simulink model "Three_Level_Inverter"  (R2020b)
settings: Solver=VariableStepAuto  StartTime=0.0  StopTime=0.02  FixedStep=1e-9  RelTol=1e-3
values from neighbouring files (symbols this model uses):
  Tri_wave_dt = 25e-6    (= 2.5e-05)    [inv_sim.m]
  Ts = 2e-6    (= 2e-06)    [inv_sim.m]
libraries: ee_lib x55, fl_lib x36, nesl_utility x34, simulink x2
(part 1 of 2)
settings Model: Creator=ge62gas  LastModifiedBy=ge62gas

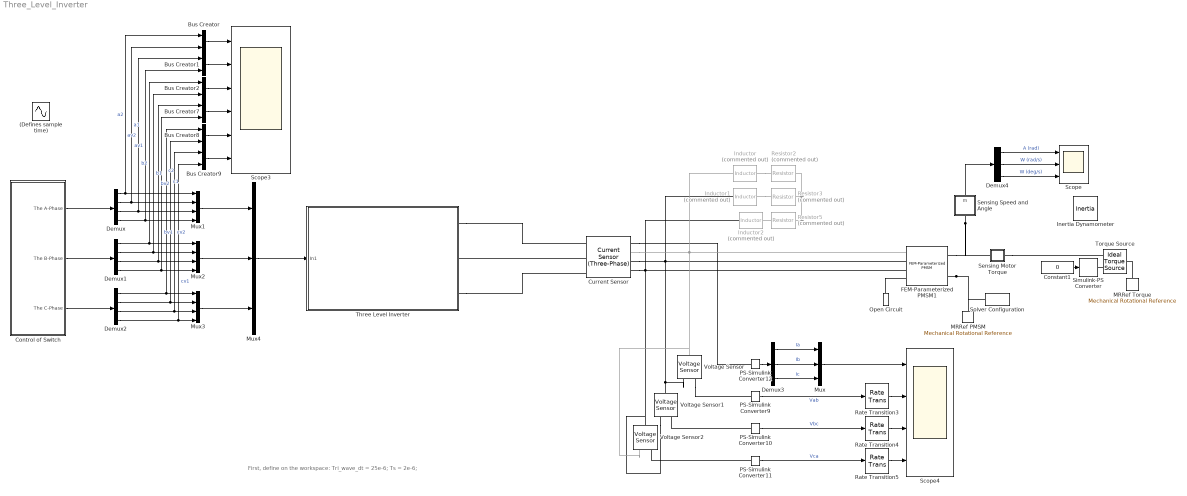
== system Three_Level_Inverter ==
  note: First, define on the workspace:
      |
      | Tri_wave_dt = 25e-6;
      | Ts = 2e-6;
  (Defines sample time) : Sin  SampleTime=Tri_wave_dt/10
  Bus Creator{,1..2,7..9} (6 alike) : BusCreator  Inputs=2
  Constant1 : Constant  Value=0
  Control of Switch : Subsystem
  Current Sensor : ee_lib/Sensors & Transducers/Current Sensor (Three-Phase)
      settings: SourceProductName=Electrical  InternalSimscapePortConfiguration="{\"Bottom\":[],\"Left\":[{\"id\":\"a1\",\"label\":\"a1\",\"type\":\"foundation.electrical.electrical\"},{\"id\":\"b1\",\"label\":\"b1\",\"type\":\"foundation.electrical.electrical\"},{\"id\":\"c1\",\"label\":\"c1\",\"type\":\"foundation.electrical.electrical\"}],\"Right\":[{\"id\":\"I_output\",\"label\":\"I\",\"type\":\"output\"},{\"id\":\"a2\",\"label\":\"a2\",\"type\":\"foundation.electrical.electrical\"},{\"id\":\"b2\",\"label\":\"b2\",\"type\":\"foundation.electrical.electrical\"},{\"id\":\"c2\",\"label\":\"c2\",\"type\":\"foundation.electrical.electrical\"}],\"Top\":[]}"
  Demux : Demux
  Demux1 : Demux
  Demux2 : Demux
  Demux3 : Demux  Outputs=3
  Demux4 : Demux  Outputs=3
  FEM-Parameterized PMSM1 : ee_lib/Electromechanical/Permanent Magnet/FEM-Parameterized PMSM  parameterization=1  winding_type=ee.enum.statorconnection.wye  iVec=[-2, 0, 2] A  xVec=xVec rad  dfluxdiMatrix=0.0002 * ones(3, 4) Wb/A  dfluxdxMatrix=[0, -.16, .16, 0; 0, -.16, .16, 0; 0, -.16, .16, 0] Wb/rad  calculate_torque_matrix=1  TorqueMatrix=zeros(3, 3, 3, 4) N*m  idVec1=[-200, 0, 200] A  iqVec1=[-200, 0, 200] A  LdMatrix=0.0002 * ones(3, 3) H  LqMatrix=0.0002 * ones(3, 3) H  PmMatrix=0.1 * ones(3, 3) Wb  N=6  interp_method=simscape.enum.interpolation.smooth  Rs=Rs Ohm  Ms=0.00002 H  L0=0.00016 H  losses_oc=[500 1500 0] W  losses_sc=[200 600 0] W  f_losses=140 Hz  Isc_losses=350 A  Inertia=0.01 kg*m^2  lam=0 N*m/(rad/s)  i_d_specify=on  i_d_priority=High  i_d=0 A  i_d_nominal_specify=off  i_d_nominal_unit=A  i_d_nominal_value=1  i_q_specify=on  i_q_priority=High  i_q=0 A  i_q_nominal_specify=off  i_q_nominal_unit=A  i_q_nominal_value=1  torque_specify=off  torque_priority=None  torque=0 N*m  torque_nominal_specify=off  torque_nominal_unit=N*m  torque_nominal_value=1  angular_velocity_specify=on  angular_velocity_priority=High  angular_velocity=3000 deg/s  angular_velocity_nominal_specify=off  angular_velocity_nominal_unit=rpm  angular_velocity_nominal_value=1  angular_position_specify=on  angular_position_priority=High  angular_position=11 deg  angular_position_nominal_specify=off  angular_position_nominal_unit=deg  angular_position_nominal_value=1  Tmeas=298.15 K  alpha=3.93e-3 1/K  alpha_flux=-0.001 1/K  stator_thermal_mass=100 J/K  stator_initial_temperatures=[298.15, 298.15, 298.15] K  rotor_thermal_mass=200 J/K  rotor_initial_temperature=298.15 K  Rm_percent_rotor=90  Rd_percent_rotor=30  idVec=idVec A  iqVec=iqVec A  dfluxAdiaMatrix3D=dfluxAdiaMatrix Wb/A  dfluxAdibMatrix3D=dfluxAdibMatrix Wb/A  dfluxAdicMatrix3D=dfluxAdicMatrix Wb/A  dfluxAdxMatrix3D=dfluxAdxMatrix Wb/rad  TorqueMatrix3D=TorqueMatrix N*m  iaVec=[-200, 0, 200] A  ibVec=[-200, 0, 200] A  icVec=[-200, 0, 200] A  dfluxAdiaMatrix=zeros(3, 3, 3, 4) Wb/A  dfluxAdibMatrix=zeros(3, 3, 3, 4) Wb/A  dfluxAdicMatrix=zeros(3, 3, 3, 4) Wb/A  dfluxAdxMatrix=zeros(3, 3, 3, 4) Wb/rad  param_dq0=1  winding_type_dq0=1  nPolePairs=4  parks_type=1  idVec2=[-200, 0, 200] A  iqVec2=[-200, 0, 200] A  magVec2=[0, 100, 200] A  betaVec2=[-180, -90, 0, 90, 180] deg  xVec2=[0, 5, 10, 15, 20, 25, 30] deg  fluxD_dq0=zeros(3, 3, 7) Wb  fluxQ_dq0=zeros(3, 3, 7) Wb  fluxA_dq0=zeros(3, 3, 7) Wb  Torque_dq0=zeros(3, 3, 7) N*m  fluxD_IBX=zeros(3, 5, 7) Wb  fluxQ_IBX=zeros(3, 5, 7) Wb  fluxA_IBX=zeros(3, 5, 7) Wb  Torque_IBX=zeros(3, 5, 7) N*m
      settings: SourceProductName=Electrical  LogSimulationData=on  InternalSimscapePortConfiguration="{\"Bottom\":[],\"Left\":[{\"id\":\"a\",\"label\":\"a\",\"type\":\"foundation.electrical.electrical\"},{\"id\":\"b\",\"label\":\"b\",\"type\":\"foundation.electrical.electrical\"},{\"id\":\"c\",\"label\":\"c\",\"type\":\"foundation.electrical.electrical\"},{\"id\":\"n\",\"label\":\"n\",\"type\":\"foundation.electrical.electrical\"}],\"Right\":[{\"id\":\"R\",\"label\":\"R\",\"type\":\"foundation.mechanical.rotational.rotational\"},{\"id\":\"C\",\"label\":\"C\",\"type\":\"foundation.mechanical.rotational.rotational\"}],\"Top\":[]}"
  Inductor : ee_lib/Passive/Inductor  Commented=on  l=1e-3 H  L_tol=20  enable_L_tol=0  tol_distribution=1  nSigma=4  r=0 Ohm  g=1e-9 1/Ohm  enable_operating_limits=0  operating_limit_action=2  max_working_current=1 A  power_rating=1 W  enable_faults=0  fault_action=1  lambdaPercent=50  k_faulted=0.9999  turnsShort=0  openCct=0  groundShort=0  groundShortG=0 1/Ohm  tau_fault=1e-3 s  enable_temporal_fault=0  t_fault=1 s  enable_behavioral_fault=0  max_permissible_voltage=100 V  n_fail_on_voltage=1  max_permissible_current=1 A  t_fail_on_current=1 s  i_L_specify=on  i_L_priority=High  i_L=-26 A  i_L_nominal_specify=off  i_L_nominal_unit=A  i_L_nominal_value=1
  Inductor1 : ee_lib/Passive/Inductor  Commented=on  l=1e-3 H  L_tol=20  enable_L_tol=0  tol_distribution=1  nSigma=4  r=0 Ohm  g=1e-9 1/Ohm  enable_operating_limits=0  operating_limit_action=2  max_working_current=1 A  power_rating=1 W  enable_faults=0  fault_action=1  lambdaPercent=50  k_faulted=0.9999  turnsShort=0  openCct=0  groundShort=0  groundShortG=0 1/Ohm  tau_fault=1e-3 s  enable_temporal_fault=0  t_fault=1 s  enable_behavioral_fault=0  max_permissible_voltage=100 V  n_fail_on_voltage=1  max_permissible_current=1 A  t_fail_on_current=1 s  i_L_specify=on  i_L_priority=High  i_L=87.5 A  i_L_nominal_specify=off  i_L_nominal_unit=A  i_L_nominal_value=1
  Inductor2 : ee_lib/Passive/Inductor  Commented=on  l=1e-3 H  L_tol=20  enable_L_tol=0  tol_distribution=1  nSigma=4  r=0 Ohm  g=1e-9 1/Ohm  enable_operating_limits=0  operating_limit_action=2  max_working_current=1 A  power_rating=1 W  enable_faults=0  fault_action=1  lambdaPercent=50  k_faulted=0.9999  turnsShort=0  openCct=0  groundShort=0  groundShortG=0 1/Ohm  tau_fault=1e-3 s  enable_temporal_fault=0  t_fault=1 s  enable_behavioral_fault=0  max_permissible_voltage=100 V  n_fail_on_voltage=1  max_permissible_current=1 A  t_fail_on_current=1 s  i_L_specify=on  i_L_priority=High  i_L=-61.5 A  i_L_nominal_specify=off  i_L_nominal_unit=A  i_L_nominal_value=1
  Inertia Dynamometer : fl_lib/Mechanical/Rotational Elements/Inertia  inertia=1 kg*m^2  num_ports=foundation.enum.numPorts2.one  w_specify=on  w_priority=High  w=rpm0 rpm  w_nominal_specify=off  w_nominal_unit=rad/s  w_nominal_value=1  t_specify=off  t_priority=High  t=0 N*m  t_nominal_specify=off  t_nominal_unit=N*m  t_nominal_value=1
      settings: SourceProductName=Foundation Library
  MRRef PMSM : fl_lib/Mechanical/Rotational Elements/Mechanical Rotational Reference
      settings: SourceProductName=Foundation Library
  MRRef Torque : fl_lib/Mechanical/Rotational Elements/Mechanical Rotational Reference
      settings: SourceProductName=Foundation Library
  Mux : Mux  Inputs=3
  Mux1 : Mux
  Mux2 : Mux
  Mux3 : Mux
  Mux4 : Mux  Inputs=3
  Open Circuit : fl_lib/Electrical/Electrical Elements/Open Circuit  v_specify=off  v_priority=None  v=0 V  v_nominal_specify=off  v_nominal_unit=V  v_nominal_value=1
      settings: SourceProductName=Foundation Library
  PS-Simulink Converter10 : nesl_utility/PS-Simulink Converter  PhysicalDomain=network_engine_domain  SubClassName=ps_output  LeftPortType=input  RightPortType=output  PseudoPeriodic=off  Frequencies=[]  Unit=V  AffineConversion=off
      settings: SourceProductName=Utilities
  PS-Simulink Converter11 : nesl_utility/PS-Simulink Converter  PhysicalDomain=network_engine_domain  SubClassName=ps_output  LeftPortType=input  RightPortType=output  PseudoPeriodic=off  Frequencies=[]  Unit=V  AffineConversion=off
      settings: SourceProductName=Utilities
  PS-Simulink Converter12 : nesl_utility/PS-Simulink Converter  PhysicalDomain=network_engine_domain  SubClassName=ps_output  LeftPortType=input  RightPortType=output  PseudoPeriodic=off  Frequencies=[]  Unit=A  AffineConversion=off
      settings: SourceProductName=Utilities
  PS-Simulink Converter9 : nesl_utility/PS-Simulink Converter  PhysicalDomain=network_engine_domain  SubClassName=ps_output  LeftPortType=input  RightPortType=output  PseudoPeriodic=off  Frequencies=[]  Unit=V  AffineConversion=off
      settings: SourceProductName=Utilities
  Rate Transition3 : RateTransition  OutPortSampleTime=Tri_wave_dt/100
  Rate Transition4 : RateTransition  OutPortSampleTime=Tri_wave_dt/100
  Rate Transition5 : RateTransition  OutPortSampleTime=Tri_wave_dt/100
  Resistor2 : ee_lib/Passive/Resistor  Commented=on  R=1 Ohm  R_tol=5  enable_R_tol=0  tol_distribution=1  nSigma=4  enable_operating_limits=0  operating_limit_action=2  max_working_voltage=100 V  power_rating=1 W  enable_faults=0  fault_action=1  R_faulted=inf Ohm  enable_temporal_fault=0  t_fault=1 s  enable_behavioral_fault=0  max_permissible_current=1 A  t_fail_on_current=1 s  noise_mode=0  sample_time=1e-3 s  repeatability=1  auto_seed=4136433779  user_seed=0  Tdevice=25 degC  alpha=3.93e-3 1/K  Tmeas=25 degC  thermal_mass=100 J/K  power_derating_T1=70 degC  power_derating_T2=155 degC  operating_temperature_range_vec=[-50, 150] degC  temperature_specify=off  temperature_priority=High  temperature=298.15 K  temperature_nominal_specify=off  temperature_nominal_unit=K  temperature_nominal_value=1
  Resistor3 : ee_lib/Passive/Resistor  Commented=on  R=1 Ohm  R_tol=5  enable_R_tol=0  tol_distribution=1  nSigma=4  enable_operating_limits=0  operating_limit_action=2  max_working_voltage=100 V  power_rating=1 W  enable_faults=0  fault_action=1  R_faulted=inf Ohm  enable_temporal_fault=0  t_fault=1 s  enable_behavioral_fault=0  max_permissible_current=1 A  t_fail_on_current=1 s  noise_mode=0  sample_time=1e-3 s  repeatability=1  auto_seed=2348512679  user_seed=0  Tdevice=25 degC  alpha=3.93e-3 1/K  Tmeas=25 degC  thermal_mass=100 J/K  power_derating_T1=70 degC  power_derating_T2=155 degC  operating_temperature_range_vec=[-50, 150] degC  temperature_specify=off  temperature_priority=High  temperature=298.15 K  temperature_nominal_specify=off  temperature_nominal_unit=K  temperature_nominal_value=1
  Resistor5 : ee_lib/Passive/Resistor  Commented=on  R=1 Ohm  R_tol=5  enable_R_tol=0  tol_distribution=1  nSigma=4  enable_operating_limits=0  operating_limit_action=2  max_working_voltage=100 V  power_rating=1 W  enable_faults=0  fault_action=1  R_faulted=inf Ohm  enable_temporal_fault=0  t_fault=1 s  enable_behavioral_fault=0  max_permissible_current=1 A  t_fail_on_current=1 s  noise_mode=0  sample_time=1e-3 s  repeatability=1  auto_seed=994690317  user_seed=0  Tdevice=25 degC  alpha=3.93e-3 1/K  Tmeas=25 degC  thermal_mass=100 J/K  power_derating_T1=70 degC  power_derating_T2=155 degC  operating_temperature_range_vec=[-50, 150] degC  temperature_specify=off  temperature_priority=High  temperature=298.15 K  temperature_nominal_specify=off  temperature_nominal_unit=K  temperature_nominal_value=1
  Scope : Scope  NumInputPorts=3
  Scope3 : Scope  NumInputPorts=6
  Scope4 : Scope  NumInputPorts=4
  Sensing Motor Torque : Subsystem
      mask Display: disp('trq');
  Sensing Speed and Angle : Subsystem
      mask Display: disp('m')
  Simulink-PS Converter : nesl_utility/Simulink-PS Converter  PhysicalDomain=network_engine_domain  SubClassName=ps_input  LeftPortType=input  RightPortType=output  PseudoPeriodic=off  Frequencies=[]  NoiseDistribution=none  NoiseParameters=[]  Unit=N*m  AffineConversion=off  FilteringAndDerivatives=zero  SimscapeFilterOrder=1  InputFilterTimeConstant=0.001  UdotUserProvided=1
      settings: SourceProductName=Utilities
  Solver Configuration : nesl_utility/Solver Configuration  PhysicalDomain=network_engine_domain  SubClassName=solver  LeftPortType=input  RightPortType=generic  Tones=[]  Harmonics=[]  SimulateNoise=off  Profile=off  UseLocalSampling=off  EnableSwitchedLinearOptims=on  FrequencyDomain=off  UseCCode=off  RelTol=0.001  AbsTol=1e-06  MinStep=1e-09  ToWorkspace=off  RevertToSquareIcSolve=off  NumHomotopyIterations=100  PhasorMode=off  PhasorModeNumHarmonics=1  DoDC=off  ResidualTolerance=1e-9  UseLocalSolver=off  LocalSolverChoice=NE_BACKWARD_EULER_ADVANCER  LocalSolverSampleTime=Ts/1000  DoFixedCost=on  MaxNonlinIter=4  MaxModeIter=2  ComputeImpulses=off  ImpulseIterations=2  LinearAlgebra=auto  EquationFormulation=NE_TIME_EF  DelaysMemoryBudget=1024  AutomaticFiltering=on  FilteringTimeConstant=0.001  PartitionStorageMethod=AS_NEEDED  PartitionMemoryBudget=1024  PartitionMethod=FAST
      settings: SourceProductName=Utilities
  Three Level Inverter : Subsystem
  Torque Source : fl_lib/Mechanical/Mechanical Sources/Ideal Torque Source
      settings: SourceProductName=Foundation Library
  Voltage Sensor : fl_lib/Electrical/Electrical Sensors/Voltage Sensor
  Voltage Sensor1 : fl_lib/Electrical/Electrical Sensors/Voltage Sensor
  Voltage Sensor2 : fl_lib/Electrical/Electrical Sensors/Voltage Sensor
  wires:
  Control of Switch/3(The C-Phase) -> Demux2/1
  Control of Switch/2(The B-Phase) -> Demux1/1
  Bus Creator1/1 -> Scope3/2
  Bus Creator2/1 -> Scope3/3
  Bus Creator/1 -> Scope3/1
  Control of Switch/1(The A-Phase) -> Demux/1
  PS-Simulink Converter9/1 -> Rate Transition3/1  "Vab"
  PS-Simulink Converter10/1 -> Rate Transition4/1  "Vbc"
  PS-Simulink Converter11/1 -> Rate Transition5/1  "Vca"
  Demux/4 -> Mux1/4, Bus Creator1/2  "av1"
  Demux/1 -> Mux1/1, Bus Creator/1  "a2"
  Demux/2 -> Mux1/2, Bus Creator/2  "a1"
  Demux/3 -> Mux1/3, Bus Creator1/1  "av2"
  Bus Creator7/1 -> Scope3/4
  Bus Creator9/1 -> Scope3/6
  Bus Creator8/1 -> Scope3/5
  Demux1/1 -> Mux2/1, Bus Creator2/1  "b2"
  Demux1/4 -> Mux2/4, Bus Creator7/2  "bv1"
  Demux2/1 -> Mux3/1, Bus Creator8/1  "c2"
  Demux1/3 -> Mux2/3, Bus Creator7/1  "bv2"
  Demux2/4 -> Mux3/4, Bus Creator9/2  "cv1"
  Demux1/2 -> Mux2/2, Bus Creator2/2  "b1"
  Demux2/2 -> Mux3/2, Bus Creator8/2  "c1"
  Demux2/3 -> Mux3/3, Bus Creator9/1  "cv2"
  Demux3/1 -> Mux/1  "Ia"
  Demux3/2 -> Mux/2  "Ib"
  Demux3/3 -> Mux/3  "Ic"
  PS-Simulink Converter12/1 -> Demux3/1
  Mux/1 -> Scope4/1
  Rate Transition4/1 -> Scope4/3
  Rate Transition3/1 -> Scope4/2
  Rate Transition5/1 -> Scope4/4
  Mux1/1 -> Mux4/1
  Mux2/1 -> Mux4/2
  Mux3/1 -> Mux4/3
  Mux4/1 -> Three Level Inverter/1(In1)
  Constant1/1 -> Simulink-PS Converter/1
  Demux4/1 -> Scope/1  "A (rad)"
  Demux4/2 -> Scope/2  "W (rad/s)"
  Sensing Speed and Angle/1(m) -> Demux4/1
  Demux4/3 -> Scope/3  "W (deg/s)"
  connections:
  Voltage Sensor1/RConn2 -- Voltage Sensor2/LConn1 -- FEM-Parameterized PMSM1/LConn3 -- Current Sensor/RConn4 -- Inductor2/LConn1
  Inductor1/RConn1 -- Resistor3/LConn1
  Inductor/RConn1 -- Resistor2/LConn1
  Resistor5/LConn1 -- Inductor2/RConn1
  Voltage Sensor/RConn1 -- PS-Simulink Converter9/LConn1
  PS-Simulink Converter10/LConn1 -- Voltage Sensor1/RConn1
  PS-Simulink Converter11/LConn1 -- Voltage Sensor2/RConn1
  Current Sensor/RConn1 -- PS-Simulink Converter12/LConn1
  Resistor5/RConn1 -- Resistor2/RConn1 -- Resistor3/RConn1
  Sensing Speed and Angle/LConn1 -- Sensing Motor Torque/LConn1 -- FEM-Parameterized PMSM1/RConn1
  Sensing Motor Torque/RConn1 -- Torque Source/RConn2
  FEM-Parameterized PMSM1/RConn2 -- MRRef PMSM/LConn1 -- Solver Configuration/RConn1
  MRRef Torque/LConn1 -- Torque Source/LConn1
  Open Circuit/LConn1 -- FEM-Parameterized PMSM1/LConn4
  Three Level Inverter/RConn1 -- Current Sensor/LConn1
  Current Sensor/LConn2 -- Three Level Inverter/RConn2
  Three Level Inverter/RConn3 -- Current Sensor/LConn3
  Simulink-PS Converter/RConn1 -- Torque Source/RConn1
  Voltage Sensor/RConn2 -- Voltage Sensor1/LConn1 -- FEM-Parameterized PMSM1/LConn2 -- Current Sensor/RConn3 -- Inductor1/LConn1
  Inductor/LConn1 -- FEM-Parameterized PMSM1/LConn1 -- Current Sensor/RConn2 -- Voltage Sensor2/RConn2 -- Voltage Sensor/LConn1

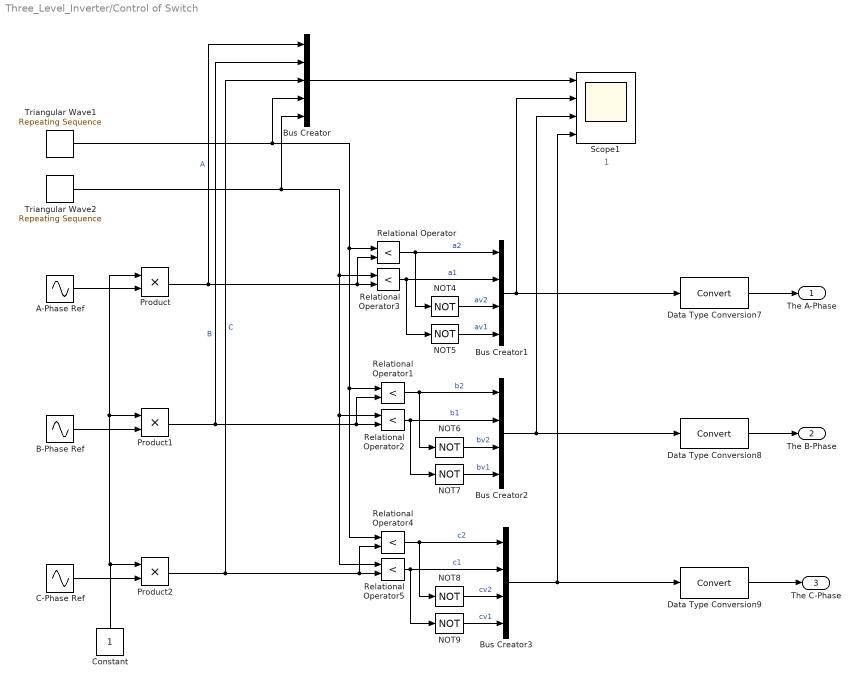
== system Three_Level_Inverter/Control of Switch ==
  note: 1
  A-Phase Ref : Sin  Frequency=2*pi*50  Phase=pi  SampleTime=0
  B-Phase Ref : Sin  Frequency=2*pi*50  Phase=pi-2*pi/3  SampleTime=0
  Bus Creator : BusCreator  Inputs=5
  Bus Creator1 : BusCreator  Inputs=4
  Bus Creator2 : BusCreator  Inputs=4
  Bus Creator3 : BusCreator  Inputs=4
  C-Phase Ref : Sin  Frequency=2*pi*50  Phase=pi+2*pi/3  SampleTime=0
  Constant : Constant
  Data Type Conversion7 : DataTypeConversion
  Data Type Conversion8 : DataTypeConversion
  Data Type Conversion9 : DataTypeConversion
  NOT{4..9} (6 alike) : Logic  Operator=NOT  IconShape=distinctive  AllPortsSameDT=off  OutDataTypeStr=boolean
  Product : Product
  Product1 : Product
  Product2 : Product
  Relational Operator{,1..5} (6 alike) : RelationalOperator  Operator=<  OutDataTypeStr=boolean  RndMeth=Simplest
  Scope1 : Scope  NumInputPorts=4
  Triangular Wave1 : simulink/Sources/Repeating Sequence  rep_seq_t=[0 Tri_wave_dt 2*Tri_wave_dt]  rep_seq_y=[0 1 0]
  Triangular Wave2 : simulink/Sources/Repeating Sequence  rep_seq_t=[0 Tri_wave_dt 2*Tri_wave_dt]  rep_seq_y=[0 -1 0]
  The A-Phase : Outport
  The B-Phase : Outport  Port=2
  The C-Phase : Outport  Port=3
  wires:
  Bus Creator/1 -> Scope1/1
  A-Phase Ref/1 -> Product/2
  Constant/1 -> Product/1, Product1/1, Product2/1
  B-Phase Ref/1 -> Product1/2
  C-Phase Ref/1 -> Product2/2
  Product1/1 -> Bus Creator/2, Relational Operator1/2, Relational Operator2/2  "B"
  Relational Operator/1 -> NOT4/1, Bus Creator1/1  "a2"
  Product/1 -> Bus Creator/1, Relational Operator/2, Relational Operator3/2  "A"
  Bus Creator2/1 -> Scope1/3, Data Type Conversion8/1
  Bus Creator1/1 -> Scope1/2, Data Type Conversion7/1
  Data Type Conversion9/1 -> The C-Phase/1
  Data Type Conversion8/1 -> The B-Phase/1
  Data Type Conversion7/1 -> The A-Phase/1
  Relational Operator3/1 -> NOT5/1, Bus Creator1/2  "a1"
  NOT6/1 -> Bus Creator2/3  "bv2"
  Bus Creator3/1 -> Scope1/4, Data Type Conversion9/1
  NOT4/1 -> Bus Creator1/3  "av2"
  NOT5/1 -> Bus Creator1/4  "av1"
  Relational Operator5/1 -> Bus Creator3/2, NOT9/1  "c1"
  Triangular Wave1/1 -> Bus Creator/4, Relational Operator1/1, Relational Operator4/1, Relational Operator/1
  Product2/1 -> Bus Creator/3, Relational Operator4/2, Relational Operator5/2  "C"
  Relational Operator4/1 -> Bus Creator3/1, NOT8/1  "c2"
  NOT8/1 -> Bus Creator3/3  "cv2"
  NOT9/1 -> Bus Creator3/4  "cv1"
  NOT7/1 -> Bus Creator2/4  "bv1"
  Relational Operator2/1 -> Bus Creator2/2, NOT7/1  "b1"
  Relational Operator1/1 -> Bus Creator2/1, NOT6/1  "b2"
  Triangular Wave2/1 -> Bus Creator/5, Relational Operator2/1, Relational Operator5/1, Relational Operator3/1

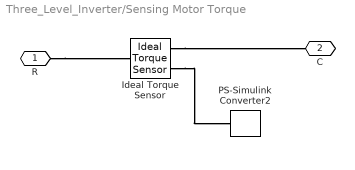
== system Three_Level_Inverter/Sensing Motor Torque ==
  Ideal Torque Sensor : fl_lib/Mechanical/Mechanical Sensors/Ideal Torque Sensor
      settings: SourceProductName=Foundation Library
  PS-Simulink Converter2 : nesl_utility/PS-Simulink Converter  PhysicalDomain=network_engine_domain  SubClassName=ps_output  LeftPortType=input  RightPortType=output  PseudoPeriodic=off  Frequencies=[]  Unit=N*m  AffineConversion=off
      settings: SourceProductName=Utilities
  R : PMIOPort  Side=Left
  C : PMIOPort  Port=2  Side=Right
  connections:
  Ideal Torque Sensor/RConn2 -- PS-Simulink Converter2/LConn1
  R/RConn1 -- Ideal Torque Sensor/LConn1
  Ideal Torque Sensor/RConn1 -- C/RConn1

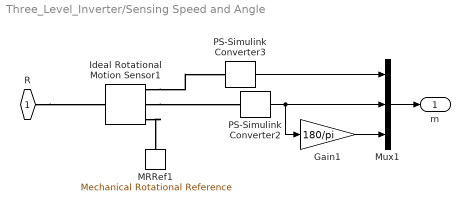
== system Three_Level_Inverter/Sensing Speed and Angle ==
  Gain1 : Gain  Gain=180/pi
  Ideal Rotational Motion Sensor1 : fl_lib/Mechanical/Mechanical Sensors/Ideal Rotational Motion Sensor  wrap_angle=simscape.enum.onoff.off  offset=0 deg
      settings: SourceProductName=Foundation Library
  MRRef1 : fl_lib/Mechanical/Rotational Elements/Mechanical Rotational Reference
      settings: SourceProductName=Foundation Library
  Mux1 : Mux  Inputs=3
  PS-Simulink Converter2 : nesl_utility/PS-Simulink Converter  PhysicalDomain=network_engine_domain  SubClassName=ps_output  LeftPortType=input  RightPortType=output  PseudoPeriodic=off  Frequencies=[]  Unit=rad/s  AffineConversion=off
      settings: SourceProductName=Utilities
  PS-Simulink Converter3 : nesl_utility/PS-Simulink Converter  PhysicalDomain=network_engine_domain  SubClassName=ps_output  LeftPortType=input  RightPortType=output  PseudoPeriodic=off  Frequencies=[]  Unit=rad  AffineConversion=off
      settings: SourceProductName=Utilities
  R : PMIOPort  Side=Left
  m : Outport  VectorParamsAs1DForOutWhenUnconnected=off
  wires:
  Mux1/1 -> m/1
  PS-Simulink Converter2/1 -> Gain1/1, Mux1/2
  PS-Simulink Converter3/1 -> Mux1/1
  Gain1/1 -> Mux1/3
  connections:
  Ideal Rotational Motion Sensor1/RConn1 -- MRRef1/LConn1
  Ideal Rotational Motion Sensor1/RConn3 -- PS-Simulink Converter3/LConn1
  Ideal Rotational Motion Sensor1/RConn2 -- PS-Simulink Converter2/LConn1
  R/RConn1 -- Ideal Rotational Motion Sensor1/LConn1
